simulink model "Ex4sim"  (R2024b)
settings: Solver=VariableStepAuto  StartTime=0.0  StopTime=3  MaxStep=1e-5  RelTol=1e-5
values from neighbouring files (symbols this model uses):
  k = acker(phi, gamma,eigs_d)    [Ex2.m]    (also in Ex3.m = dlqr(phi_e,gamma_e,Q,R); Ex4.m = acker(A_z,B_z,eigs); Extended_Estimator.m = acker(A,B,pol_c))
  Tl = 1/(2*w_gc)    (= 0.0416666666667)    [Ex1.m]    (also in Ex4.m = 1/(2*w_n); Extended_Estimator.m = 1/(2*wn))
  w = 6    [Ex4.m]    (also in Extended_Estimator.m)
settings Model: Creator=bmm1  LastModifiedBy=bmm1

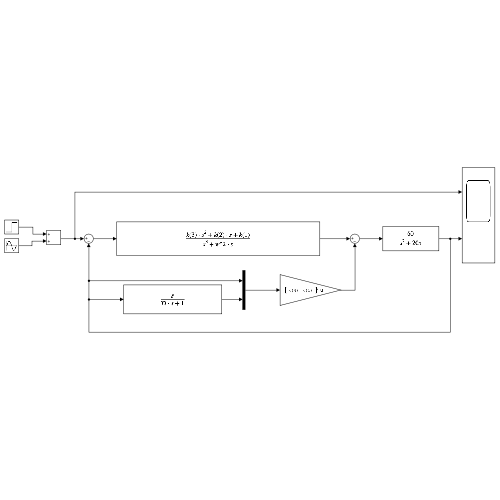
[thumbnail: Simulink's stored preview of the top-level diagram]
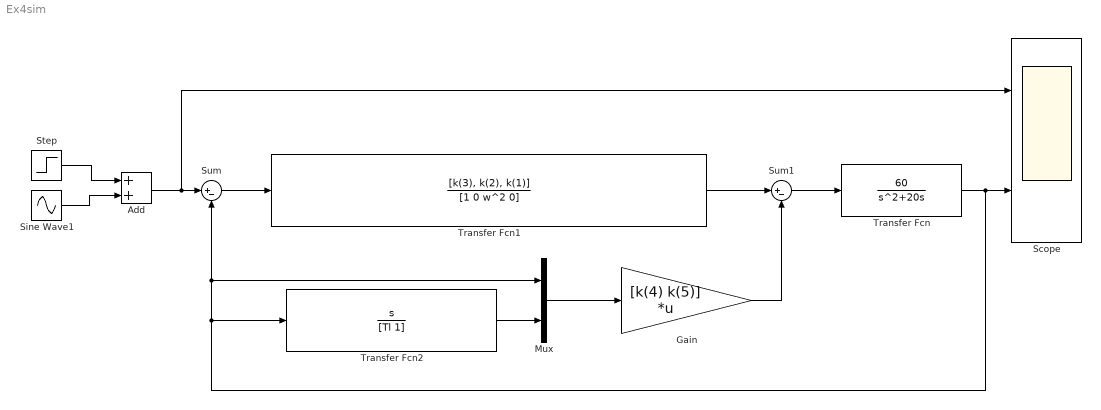
== system Ex4sim ==
  Add : Sum
  Gain : Gain  Gain=[k(4) k(5)]  Multiplication=Matrix(K*u)
  Mux : Mux  Inputs=2
  Scope : Scope  NumInputPorts=2
  Sine Wave1 : Sin  Frequency=6  SampleTime=0
  Step : Step  SampleTime=0
  Sum : Sum  Inputs=|+-
  Sum1 : Sum  Inputs=|+-
  Transfer Fcn : TransferFcn  Numerator=[60]  Denominator=[1 20 0]
  Transfer Fcn1 : TransferFcn  Numerator=[k(3), k(2), k(1)]  Denominator=[1 0 w^2 0]
  Transfer Fcn2 : TransferFcn  Numerator=[1 0]  Denominator=[Tl 1]
  wires:
  Sine Wave1/1 -> Add/2
  Sum/1 -> Transfer Fcn1/1
  Gain/1 -> Sum1/2
  Transfer Fcn/1 -> Scope/2, Sum/2, Mux/1, Transfer Fcn2/1
  Mux/1 -> Gain/1
  Transfer Fcn1/1 -> Sum1/1
  Sum1/1 -> Transfer Fcn/1
  Add/1 -> Scope/1, Sum/1
  Step/1 -> Add/1
  Transfer Fcn2/1 -> Mux/2
